simulink model "threeservos"  (Simulink 4.00)
settings: Solver=ode45  StartTime=0.0  StopTime=1  RelTol=1e-3
InitFcn:
  | clear functions
libraries: truetime x1
settings Model: Creator=anton  LastModifiedBy=anton  SaveTime=off  SaveOutput=off  LimitDataPoints=off  ExtModeTrigMode=oneshot  ExtModeArmWhenConnect=off  ExtModeAutoUpdateStatusClock=off  BlockReductionOpt=off

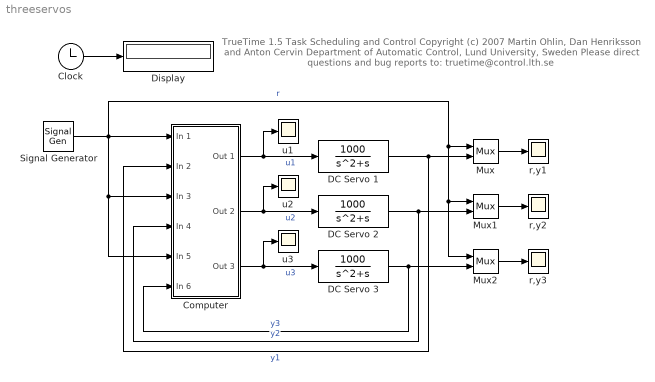
== system threeservos ==
  note: TrueTime 1.5  Task Scheduling and Control
      | Copyright (c) 2007
      | Martin Ohlin, Dan Henriksson and Anton Cervin
      | Department of Automatic Control, Lund University, Sweden
      | Please direct questions and bug reports to:  truetime@control.lth.se
  Clock : Clock
      settings: DisplayTime=off  Decimation=10
  Computer : Subsystem
      settings: RTWFcnNameOpts=Auto  RTWFileNameOpts=Auto
  DC Servo 1 : TransferFcn  Numerator=[1000]  Denominator=[1 1 0]  AbsoluteTolerance=auto  Realization=auto
  DC Servo 2 : TransferFcn  Numerator=[1000]  Denominator=[1 1 0]  AbsoluteTolerance=auto  Realization=auto
  DC Servo 3 : TransferFcn  Numerator=[1000]  Denominator=[1 1 0]  AbsoluteTolerance=auto  Realization=auto
  Display : Display
      settings: Format=short
  Mux : Mux  Inputs=2
      settings: DisplayOption=none
  Mux1 : Mux  Inputs=2
      settings: DisplayOption=none
  Mux2 : Mux  Inputs=2
      settings: DisplayOption=none
  Signal Generator : SignalGenerator  WaveForm=square  Amplitude=1  Frequency=1  Units=Hertz
  r,y1 : Scope
      settings: TimeRange=1  YMin=-2  YMax=2  SaveToWorkspace=off  SaveName=ry1  MaxDataPoints=5000
  r,y2 : Scope
      settings: TimeRange=1  YMin=-2  YMax=2  SaveToWorkspace=off  SaveName=ry2  MaxDataPoints=5000
  r,y3 : Scope
      settings: TimeRange=1  YMin=-2  YMax=2  SaveToWorkspace=off  SaveName=ry3  MaxDataPoints=5000
  u1 : Scope
      settings: TimeRange=1  YMin=-2  YMax=2  SaveToWorkspace=off  SaveName=ScopeData  MaxDataPoints=5000
  u2 : Scope
      settings: TimeRange=1  YMin=-2  YMax=2  SaveToWorkspace=off  SaveName=ScopeData  MaxDataPoints=5000
  u3 : Scope
      settings: TimeRange=1  YMin=-2  YMax=2  SaveToWorkspace=off  SaveName=ScopeData  MaxDataPoints=5000
  wires:
  Clock/1 -> Display/1
  Computer/1(Out 1) -> DC Servo 1/1, u1/1  "u1"
  Signal Generator/1 -> Computer/3(In 3), Computer/5(In 5), Computer/1(In 1), Mux/1, Mux1/1, Mux2/1  "r"
  Computer/2(Out 2) -> DC Servo 2/1, u2/1  "u2"
  Computer/3(Out 3) -> DC Servo 3/1, u3/1  "u3"
  DC Servo 1/1 -> Computer/2(In 2), Mux/2  "y1"
  DC Servo 2/1 -> Computer/4(In 4), Mux1/2  "y2"
  DC Servo 3/1 -> Computer/6(In 6), Mux2/2  "y3"
  Mux/1 -> r,y1/1
  Mux1/1 -> r,y2/1
  Mux2/1 -> r,y3/1

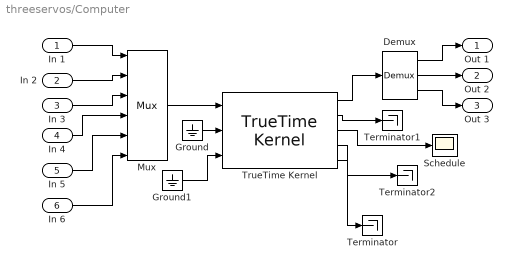
== system threeservos/Computer ==
  In 1 : Inport  Port=1  LatchInput=off
  In 2 : Inport  Port=2  LatchInput=off
  In 3 : Inport  Port=3  LatchInput=off
  In 4 : Inport  Port=4  LatchInput=off
  In 5 : Inport  Port=5  LatchInput=off
  In 6 : Inport  Port=6  LatchInput=off
  Demux : Demux  Outputs=3  BusSelectionMode=off
  Ground : Ground
  Ground1 : Ground
  Mux : Mux  Inputs=6
      settings: DisplayOption=none
  Schedule : Scope
      settings: TickLabels=on  TimeRange=1  YMin=0.8  YMax=3.7  SaveToWorkspace=off  SaveName=schedule  MaxDataPoints=5000
  Terminator : Terminator
  Terminator1 : Terminator
  Terminator2 : Terminator
  TrueTime Kernel : truetime/TrueTime Kernel  sfun=threeservos_init  args=0  battery=off  clockdrift=0  clockoffset=0
  Out 1 : Outport  Port=1
  Out 2 : Outport  Port=2
  Out 3 : Outport  Port=3
  wires:
  Mux/1 -> TrueTime Kernel/1
  Demux/1 -> Out 1/1
  TrueTime Kernel/1 -> Demux/1
  In 1/1 -> Mux/1
  In 2/1 -> Mux/2
  In 3/1 -> Mux/3
  In 4/1 -> Mux/4
  In 5/1 -> Mux/5
  In 6/1 -> Mux/6
  Demux/2 -> Out 2/1
  Demux/3 -> Out 3/1
  TrueTime Kernel/3 -> Schedule/1
  TrueTime Kernel/4 -> Terminator2/1
  TrueTime Kernel/2 -> Terminator1/1
  Ground/1 -> TrueTime Kernel/2
  Ground1/1 -> TrueTime Kernel/3
  TrueTime Kernel/5 -> Terminator/1
